simulink model "DC_DC_Chopper"  (R2016b)
settings: Solver=ode23t  StartTime=0.0  StopTime=0.002  MaxStep=1.e-06  MinStep=1.e-08  RelTol=1e-3  EnableMultiTasking=on
libraries: powerlib x8, simulink x1
settings Model: Creator=sc  LastModifiedBy=Osman Kukrer
settings SolverCC: InitialStep=1.e-07
settings DataIOCC: LimitDataPoints=on  SaveFormat=Array  SignalLoggingSaveFormat=ModelDataLogs
settings OptimizationCC: ExpressionDepthLimit=2147483647  InitFltsAndDblsToZero=on  LifeSpan=inf
settings DebuggingCC: UnderspecifiedInitializationDetection=Classic  MergeDetectMultiDrivingBlocksExec=none  SolverPrmCheckMsg=warning  FcnCallInpInsideContextMsg=warning  ModelReferenceIOMismatchMessage=error  StateNameClashWarn=warning  SFUnexpectedBacktrackingDiag=warning  SFNoUnconditionalDefaultTransitionDiag=warning  SFExecutionAtInitializationDiag=none
settings HardwareCC: ProdBitPerPointer=32  ProdBitPerSizeT=32  ProdBitPerPtrDiffT=32  ProdLargestAtomicFloat=None  ProdIntDivRoundTo=Undefined  ProdEndianess=Unspecified  ProdWordSize=32  ProdHWDeviceType=32-bit Generic
settings ModelReferenceCC: PropagateSignalLabelsOutOfModel=off
settings GRTTargetCC: TargetLangStandard=C89/C90 (ANSI)  CombineOutputUpdateFcns=off  GRTInterface=on
settings ConfigComp: CovMetricSettings=dw  CovHtmlReporting=on  CovSaveCumulativeToWorkspaceVar=on  CovSaveSingleToWorkspaceVar=on  CovExternalEMLEnable=off

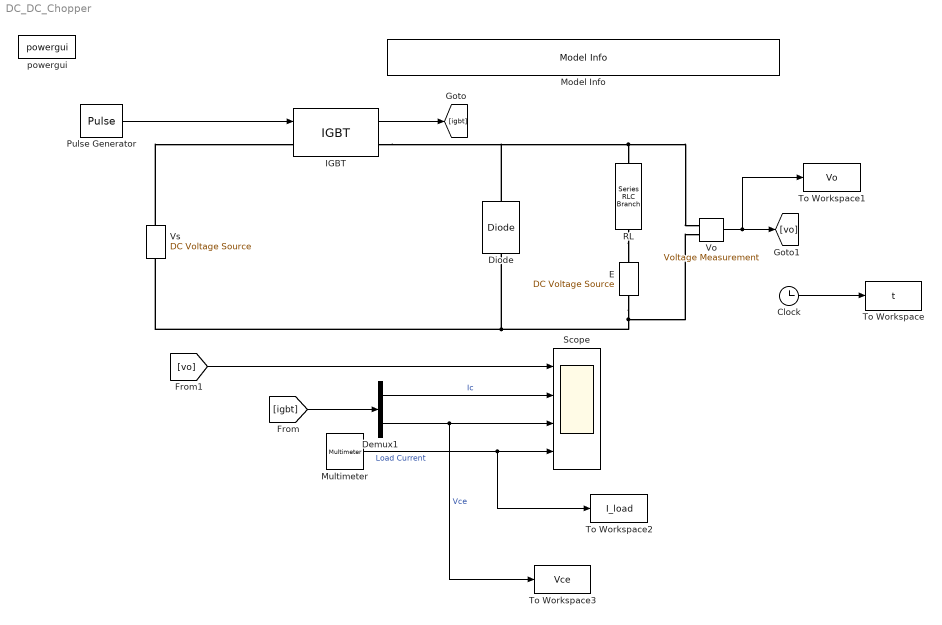
== system DC_DC_Chopper ==
  " RL" : powerlib/Elements/Series RLC Branch  LConnTagsString=__new0  RConnTagsString=__new0  BranchType=RL  Resistance=5  Inductance=5e-3  SetiL0=off  InitialCurrent=0  Capacitance=1.0  Setx0=off  InitialVoltage=0  Measurements=Branch current
  Clock : Clock
  Demux1 : Demux  Outputs=2
  Diode : powerlib/Power Electronics/Diode  Ron=0.001  Lon=0  Vf=0.7  IC=0  UseSnubber=off  Rs=inf  Cs=250e-9  Measurements=off
  E : powerlib/Electrical Sources/DC Voltage Source  Amplitude=80  Measurements=None
  IGBT : powerlib/Power Electronics/IGBT  Ron=0.001  Lon=0  Vf=1  Tf=1e-6  Tt=2e-6  IC=0  Rs=5000  Cs=1.e-5  Measurements=on
  Model Info : simulink/Model-Wide Utilities/Model Info  BlockCM=None  Frame=on  DisplayStringWithTags=DC-DC Chopper (DC-DC Step-down converter)  HorizontalTextAlignment=Center  LeftAlignmentValue=0.5  SourceBlockDiagram=DC_DC_Chopper  TagMaxNumber=20
  Multimeter : powerlib/Measurements/Multimeter  PhasorSimulation=off  OutputType=Complex  sel=1  L=1  Gain=1  yselected="{'Ib:  RL'};"  PSBOutputType=1  PSBequivalent=0  AxesSetting=[0,0.1,-100,100]  Display=1  SavedBlockNames=-11
  Pulse Generator : DiscretePulseGenerator  PulseType=Time based  Period=2.e-04  PulseWidth=40
  Scope : Scope  NumInputPorts=4
  To Workspace : ToWorkspace  VariableName=t  SampleTime=-1
  To Workspace1 : ToWorkspace  VariableName=Vo  SampleTime=-1
  To Workspace2 : ToWorkspace  VariableName=I_load  SampleTime=-1
  To Workspace3 : ToWorkspace  VariableName=Vce  SampleTime=-1
  Vo : powerlib/Measurements/Voltage Measurement  PhasorSimulation=off  OutputType=Complex  PSBequivalent=0
  Vs : powerlib/Electrical Sources/DC Voltage Source  Amplitude=250  Measurements=None
  powergui : powerlib/powergui  SimulationMode=Continuous  SolverType=Tustin/Backward Euler (TBE)  SampleTime=50e-6  frequency=60  SPID=off  DisableSnubberDevices=off  DisableRonSwitches=off  DisableVfSwitches=off  SwTol=0  DisplayEquations=off  Interpol=off  ExternalGateDelay=off  methode=off  Ts=0  FunctionMessages=off  echomessages=off  HookPort=off  EnableUseOfTLC=off  x0status=blocks  frequencyindice=0  Pbase=100e6  ErrMax=1e-4  Iterations=50  UnitsV=kV  UnitsW=MW  buscounter=0  RestoreLinks=warning  ResistiveCurrentMeasurement=off  Frange=[0:2:500]  Ylog=off  Xlog=on  ShowGrid=off  save=off  variable=ZData  structure=0  ZoomFFT=on  StartTime=0.0  cycles=1  DisplayStyle=1  fundamental=60  FreqAxis=off  MaxFrequency=1000  frequencyindicesteady=1  RmsSteady=1  display=off
  wires:
  Pulse Generator/1 -> IGBT/1
  IGBT/1 -> [igbt]
  [igbt] -> Demux1/1
  Vo/1 -> [vo], To Workspace1/1
  [vo] -> Scope/1
  Demux1/1 -> Scope/2  "Ic"
  Demux1/2 -> Scope/3, To Workspace3/1  "Vce"
  Multimeter/1 -> To Workspace2/1, Scope/4  "Load Current"
  Clock/1 -> To Workspace/1
  connections:
  Vs/RConn1 -- IGBT/LConn1
  " RL"/RConn1 -- E/RConn1
  IGBT/RConn1 -- Diode/RConn1 -- " RL"/LConn1 -- Vo/LConn1
  E/LConn1 -- Vs/LConn1 -- Diode/LConn1 -- Vo/LConn2
